simulink model "First_Order_System_2"  (R2024a)
settings: Solver=VariableStepAuto  StartTime=0.0  StopTime=10.0  RelTol=1e-3
settings Model: Creator=Lenovo  LastModifiedBy=Lenovo

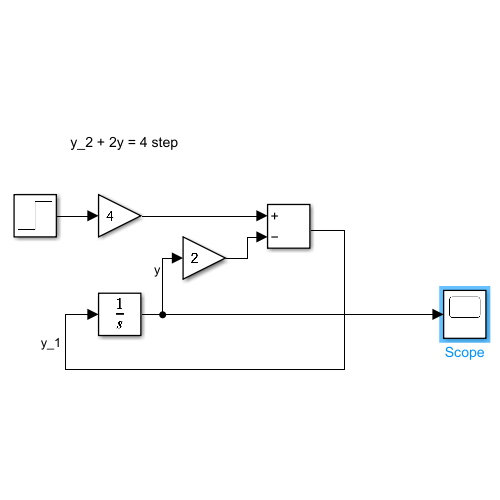
[thumbnail: Simulink's stored preview of the top-level diagram]
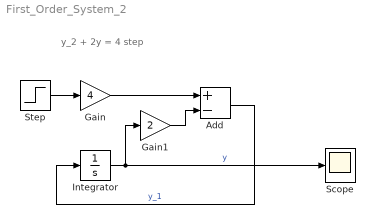
== system First_Order_System_2 ==
  note: y_2 + 2y = 4 step
  Add : Sum  Inputs=+-
  Gain : Gain  Gain=4
  Gain1 : Gain  Gain=2
  Integrator : Integrator
  Scope : Scope
  Step : Step  SampleTime=0
  wires:
  Step/1 -> Gain/1
  Add/1 -> Integrator/1  "y_1"
  Integrator/1 -> Gain1/1, Scope/1  "y"
  Gain/1 -> Add/1
  Gain1/1 -> Add/2
